simulink model "WF_offshore"  (R2024a)
settings: Solver=VariableStepAuto  StartTime=0  StopTime=1  RelTol=1e-3
values from neighbouring files (symbols this model uses):
  c_c = 0.177e-6    (= 1.77e-07)    [WF_onshore_SSO_GFL.m]    (also in WF_physical_param_offshore_supersynchronous.m = cable_220(i,6)*1e-9; WF_physical_param_onshore_SSO_020625.m = cable_220(i,6)*1e-9; initialize_params_agg.m)
  c_c_eff = c_c*n_cables    [WF_onshore_SSO_GFL.m]    (also in WF_physical_param_offshore_supersynchronous.m; WF_physical_param_onshore_SSO_020625.m; initialize_params_agg.m)
  cvtr = initialize_NR_VSC_GF(cvtr)    [NR_steadystate_VSC_GF.m]    (also in WF_onshore_SSO_GFL.m = setfield(cvtr,'parameters', p_vary.name,p_vary.val(i)); WF_physical_param_offshore_supersynchronous.m = setfield(cvtr,'parameters', p_vary.name,p_vary.val(i)); WF_physical_param_onshore_SSO_020625.m = setfield(cvtr,'parameters', p_vary.name,p_vary.val(i)); impedance_WT_blackbox.m = base_values(cvtr))
  D_C = 10:4:100    [WF_onshore_SSO_GFL.m]    (also in WF_parameter_variation.m = 10:4:150; WF_physical_param.m = 10:4:150; WF_physical_param_offshore_supersynchronous.m = 50; WF_physical_param_onshore_SSO_020625.m = 50)
  enable_pll = 1    [impedance_WT_agg.m]    (also in initialize_WT_agg.m; initialize_WT_default_gfl.m; initialize_WT_default_offshore_super.m)
  f1 = 50    [WF_onshore_SSO_GFL.m]    (also in WF_physical_param_offshore_supersynchronous.m; WF_physical_param_onshore_SSO_020625.m; initialize_params_agg.m)
  i = 1    [WF_physical_param_offshore_supersynchronous.m]    (also in WF_physical_param_onshore_SSO_020625.m)
  L = inv(R)    [participation_factors_VSC_GF.m]
  l_c = 0.386e-3    (= 0.000386)    [WF_onshore_SSO_GFL.m]    (also in WF_physical_param_offshore_supersynchronous.m = cable_220(i,5)*1e-3; WF_physical_param_onshore_SSO_020625.m = cable_220(i,5)*1e-3; initialize_params_agg.m)
  l_c_eff = l_c/n_cables    [WF_onshore_SSO_GFL.m]    (also in WF_physical_param_offshore_supersynchronous.m; WF_physical_param_onshore_SSO_020625.m; initialize_params_agg.m)
  L_comp = sqrt(2)*l_comp*(Z_b_G/(2*pi*f1))    [WF_physical_param.m]    (also in WF_physical_param_offshore_supersynchronous.m = sqrt(2)*((1/(c_c_eff/2*D_C*2*pi*f1))-(l_tf_wf*(Z_b_G)+(l_c_e; WF_physical_param_onshore_SSO_020625.m = sqrt(2)*((1/(c_c_eff/2*D_C*2*pi*f1))-(l_tf_wf*(Z_b_G)+(l_c_e; initialize_params_agg.m)
  l_OH = 0.2    [WF_onshore_SSO_GFL.m]    (also in WF_physical_param_offshore_supersynchronous.m = 0.1; WF_physical_param_onshore_SSO_020625.m = 0.1; initialize_params_agg.m = 0.1)
  l_tf_wf = tf_params(2,2)    [IM_WF_agg.m]    (also in WF_onshore_SSO_GFL.m = 0.05; WF_physical_param_offshore_supersynchronous.m = 0.05; WF_physical_param_onshore_SSO_020625.m = 0.05; initialize_params_agg.m = 0.05)
  l_tf_wt = tf_params(1,2)    [IM_WF_agg.m]    (also in WF_onshore_SSO_GFL.m = 0.0392; WF_physical_param_offshore_supersynchronous.m = 0.0392; WF_physical_param_onshore_SSO_020625.m = 0.0392; initialize_params_agg.m = 0.0392)
  Lg = p_vary(i)*((Z_b_G/(2*pi*f1)))    [WF_onshore_SSO_GFL.m]    (also in WF_physical_param_offshore_supersynchronous.m; WF_physical_param_onshore_SSO_020625.m; initialize_params_agg.m = 0.1*((Z_b_G/(2*pi*f1))))
  Lg1 = Lg    [WF_physical_param_offshore_supersynchronous.m]    (also in WF_physical_param_onshore_SSO_020625.m)
  Lg2 = Lg    [WF_physical_param_offshore_supersynchronous.m]    (also in WF_physical_param_onshore_SSO_020625.m)
  r_c = 27e-3    (= 0.027)    [WF_onshore_SSO_GFL.m]    (also in WF_physical_param_offshore_supersynchronous.m = cable_220(i,4)*1e-3; WF_physical_param_onshore_SSO_020625.m = cable_220(i,4)*1e-3; initialize_params_agg.m)
  r_c_eff = r_c/n_cables    [WF_onshore_SSO_GFL.m]    (also in WF_physical_param_offshore_supersynchronous.m; WF_physical_param_onshore_SSO_020625.m; initialize_params_agg.m)
  r_diss = .1    (= 0.1)    [WF_physical_param_offshore_supersynchronous.m]    (also in WF_physical_param_onshore_SSO_020625.m; calculate_WF.m; initialize_params_agg.m)
  r_OH = 0.02    [WF_onshore_SSO_GFL.m]    (also in WF_physical_param_offshore_supersynchronous.m = 0.01; WF_physical_param_onshore_SSO_020625.m = 0.01; initialize_params_agg.m)
  r_tf_wf = tf_params(2,1)    [IM_WF_agg.m]    (also in WF_onshore_SSO_GFL.m = 0.005; WF_physical_param_offshore_supersynchronous.m = 0.005; WF_physical_param_onshore_SSO_020625.m = 0.005; initialize_params_agg.m = 0.005)
  r_tf_wt = tf_params(1,1)    [IM_WF_agg.m]    (also in WF_onshore_SSO_GFL.m = 0.0056; WF_physical_param_offshore_supersynchronous.m = 0.0056; WF_physical_param_onshore_SSO_020625.m = 0.0056; initialize_params_agg.m = 0.0056)
  Rg = rg*Z_b_G    [WF_onshore_SSO_GFL.m]    (also in WF_physical_param_offshore_supersynchronous.m; WF_physical_param_onshore_SSO_020625.m; initialize_params_agg.m = 0.01*Z_b_G)
  Sb_WF = (3*1)*5e6    (= 15000000)    [WF_onshore_SSO_GFL.m]    (also in WF_physical_param_offshore_supersynchronous.m; WF_physical_param_onshore_SSO_020625.m; impedance_WT_blackbox.m = n_t*Sb_WT; initialize_params_agg.m = 1000000000)
  Sb_WT = 5e6    (= 5000000)    [IM_WF.m]    (also in WF_onshore_SSO_GFL.m; WF_physical_param_offshore_supersynchronous.m; WF_physical_param_onshore_SSO_020625.m; initialize_params_agg.m)
  selector_current_reference = 3    [impedance_WT_agg.m]    (also in initialize_WT_agg.m; initialize_WT_default_gfl.m; initialize_WT_default_offshore_super.m)
  selector_omega_reference = 1    [impedance_WT_agg.m]    (also in initialize_WT_agg.m; initialize_WT_default_gfl.m; initialize_WT_default_offshore_super.m)
  V_coll = 33e3    (= 33000)    [WF_onshore_SSO_GFL.m]    (also in WF_physical_param_offshore_supersynchronous.m; WF_physical_param_onshore_SSO_020625.m; initialize_params_agg.m)
  V_trans = 220e3    (= 220000)    [WF_onshore_SSO_GFL.m]    (also in WF_physical_param_offshore_supersynchronous.m; WF_physical_param_onshore_SSO_020625.m; initialize_params_agg.m)
  Z_b_G = (V_trans/sqrt(3/2))^2/Sb_WF    [WF_onshore_SSO_GFL.m]    (also in WF_physical_param_offshore_supersynchronous.m = (V_b_trans)^2/Sb_WF; WF_physical_param_onshore_SSO_020625.m = (V_b_trans)^2/Sb_WF; initialize_params_agg.m = (V_b_trans)^2/Sb_WF)
undefined symbols (not defined in the file or in its folder): opts, R
libraries: spsSeriesRLCBranchLib x105, simulink_extras x104, simulink x52, spsThreePhaseVIMeasurementLib x42, spsControlledVoltageSourceLib x42, spsGroundLib x41, spsThreePhaseTransformerTwoWindingsLib x14, powerlib_extras x13, spsVariableInductorLib x9, spsIdealSwitchLib x6, spsVariableCapacitorLib x6, spsThreePhaseSeriesRLCBranchLib x4
(part 13 of 13)

== system WF_offshore/WT_MF4/Control System/Current controller/Subsystem1 ==
  in : Inport
  Demux : Demux  Outputs=2
  Mux : Mux  Inputs=2
  Subsystem3 : Subsystem
  Subsystem6 : Subsystem
  Transfer Fcn (with initial outputs) : simulink_extras/Additional Linear/Transfer Fcn (with initial outputs)  N=[Omega]  D="[1  Omega]"  Y0=xd0  U0=xd0
  Transfer Fcn (with initial outputs)1 : simulink_extras/Additional Linear/Transfer Fcn (with initial outputs)  N=[Omega]  D="[1  Omega]"  Y0=xq0  U0=xq0
  out : Outport
  wires:
  Demux/2 -> Transfer Fcn (with initial outputs)1/1
  Demux/1 -> Transfer Fcn (with initial outputs)/1
  Subsystem3/1(x_d+ix_q) -> out/1
  in/1 -> Subsystem6/1(x_d+ix_q)
  Subsystem6/1(x_dq) -> Demux/1
  Mux/1 -> Subsystem3/1(x_dq)
  Transfer Fcn (with initial outputs)1/1 -> Mux/2
  Transfer Fcn (with initial outputs)/1 -> Mux/1

== system WF_offshore/WT_MF4/Control System/PLL1/Subsystem1 ==
  x_d+ix_q : Inport
  Complex to Real-Imag2 : ComplexToRealImag
  Mux : Mux  Inputs=2
  x_dq : Outport
  wires:
  Complex to Real-Imag2/1 -> Mux/1
  Complex to Real-Imag2/2 -> Mux/2
  Mux/1 -> x_dq/1
  x_d+ix_q/1 -> Complex to Real-Imag2/1

== system WF_offshore/WT_MF4/Control System/PLL1/Subsystem3 ==
  x_dq : Inport
  Demux : Demux  Outputs=2
  Real-Imag to Complex : RealImagToComplex
  x_d+ix_q : Outport
  wires:
  Real-Imag to Complex/1 -> x_d+ix_q/1
  x_dq/1 -> Demux/1
  Demux/2 -> Real-Imag to Complex/2
  Demux/1 -> Real-Imag to Complex/1

== system WF_offshore/WT_MF4/Control System/PQ controller/Subsystem3 ==
  x_dq : Inport
  Demux : Demux  Outputs=2
  Real-Imag to Complex : RealImagToComplex
  x_d+ix_q : Outport
  wires:
  Real-Imag to Complex/1 -> x_d+ix_q/1
  x_dq/1 -> Demux/1
  Demux/2 -> Real-Imag to Complex/2
  Demux/1 -> Real-Imag to Complex/1

== system WF_offshore/WT_MF4/Control System/Voltage controller DEM/Subsystem ==
  x : Inport
  x0 : Inport  Port=2
  Complex to Real-Imag : ComplexToRealImag
  Complex to Real-Imag1 : ComplexToRealImag
  Integrator : Integrator  InitialConditionSource=external
  Integrator1 : Integrator  InitialConditionSource=external
  Real-Imag to Complex : RealImagToComplex
  x/s : Outport
  wires:
  Integrator/1 -> Real-Imag to Complex/2
  Integrator1/1 -> Real-Imag to Complex/1
  x0/1 -> Complex to Real-Imag1/1
  Real-Imag to Complex/1 -> x/s/1
  x/1 -> Complex to Real-Imag/1
  Complex to Real-Imag1/2 -> Integrator/2
  Complex to Real-Imag1/1 -> Integrator1/2
  Complex to Real-Imag/2 -> Integrator/1
  Complex to Real-Imag/1 -> Integrator1/1

== system WF_offshore/WT_MF4/Control System/Voltage controller QSEM/Subsystem2 ==
  x_d+ix_q : Inport
  Complex to Real-Imag2 : ComplexToRealImag
  Mux : Mux  Inputs=2
  x_dq : Outport
  wires:
  Complex to Real-Imag2/1 -> Mux/1
  Complex to Real-Imag2/2 -> Mux/2
  Mux/1 -> x_dq/1
  x_d+ix_q/1 -> Complex to Real-Imag2/1

== system WF_offshore/WT_MF4/Control System/Voltage controller QSEM/Subsystem3 ==
  x_dq : Inport
  Demux : Demux  Outputs=2
  Real-Imag to Complex : RealImagToComplex
  x_d+ix_q : Outport
  wires:
  Real-Imag to Complex/1 -> x_d+ix_q/1
  x_dq/1 -> Demux/1
  Demux/2 -> Real-Imag to Complex/2
  Demux/1 -> Real-Imag to Complex/1

== system WF_offshore/WT_MF4/Control System/Voltage controller VCVSM/Subsystem ==
  x : Inport
  x0 : Inport  Port=2
  Complex to Real-Imag : ComplexToRealImag
  Complex to Real-Imag1 : ComplexToRealImag
  Integrator : Integrator  InitialConditionSource=external
  Integrator1 : Integrator  InitialConditionSource=external
  Real-Imag to Complex : RealImagToComplex
  x/s : Outport
  wires:
  Integrator/1 -> Real-Imag to Complex/2
  Integrator1/1 -> Real-Imag to Complex/1
  x0/1 -> Complex to Real-Imag1/1
  Real-Imag to Complex/1 -> x/s/1
  x/1 -> Complex to Real-Imag/1
  Complex to Real-Imag1/2 -> Integrator/2
  Complex to Real-Imag1/1 -> Integrator1/2
  Complex to Real-Imag/2 -> Integrator/1
  Complex to Real-Imag/1 -> Integrator1/1

== system WF_offshore/WT_MF5/Control System/Current controller/Subsystem ==
  x : Inport
  x0 : Inport  Port=2
  Complex to Real-Imag : ComplexToRealImag
  Complex to Real-Imag1 : ComplexToRealImag
  Integrator : Integrator  InitialConditionSource=external  AbsoluteTolerance=1e-10
  Integrator1 : Integrator  InitialConditionSource=external  AbsoluteTolerance=1e-15
  Real-Imag to Complex : RealImagToComplex
  x/s : Outport
  wires:
  Complex to Real-Imag/1 -> Integrator/1
  Complex to Real-Imag1/1 -> Integrator/2
  Complex to Real-Imag1/2 -> Integrator1/2
  x/1 -> Complex to Real-Imag/1
  Real-Imag to Complex/1 -> x/s/1
  x0/1 -> Complex to Real-Imag1/1
  Integrator1/1 -> Real-Imag to Complex/2
  Integrator/1 -> Real-Imag to Complex/1
  Complex to Real-Imag/2 -> Integrator1/1

== system WF_offshore/WT_MF5/Control System/Current controller/Subsystem1 ==
  in : Inport
  Demux : Demux  Outputs=2
  Mux : Mux  Inputs=2
  Subsystem3 : Subsystem
  Subsystem6 : Subsystem
  Transfer Fcn (with initial outputs) : simulink_extras/Additional Linear/Transfer Fcn (with initial outputs)  N=[Omega]  D="[1  Omega]"  Y0=xd0  U0=xd0
  Transfer Fcn (with initial outputs)1 : simulink_extras/Additional Linear/Transfer Fcn (with initial outputs)  N=[Omega]  D="[1  Omega]"  Y0=xq0  U0=xq0
  out : Outport
  wires:
  Transfer Fcn (with initial outputs)/1 -> Mux/1
  Transfer Fcn (with initial outputs)1/1 -> Mux/2
  Mux/1 -> Subsystem3/1(x_dq)
  Subsystem6/1(x_dq) -> Demux/1
  in/1 -> Subsystem6/1(x_d+ix_q)
  Subsystem3/1(x_d+ix_q) -> out/1
  Demux/1 -> Transfer Fcn (with initial outputs)/1
  Demux/2 -> Transfer Fcn (with initial outputs)1/1

== system WF_offshore/WT_MF5/Control System/PLL1/Subsystem1 ==
  x_d+ix_q : Inport
  Complex to Real-Imag2 : ComplexToRealImag
  Mux : Mux  Inputs=2
  x_dq : Outport
  wires:
  x_d+ix_q/1 -> Complex to Real-Imag2/1
  Mux/1 -> x_dq/1
  Complex to Real-Imag2/2 -> Mux/2
  Complex to Real-Imag2/1 -> Mux/1

== system WF_offshore/WT_MF5/Control System/PLL1/Subsystem3 ==
  x_dq : Inport
  Demux : Demux  Outputs=2
  Real-Imag to Complex : RealImagToComplex
  x_d+ix_q : Outport
  wires:
  Demux/1 -> Real-Imag to Complex/1
  Demux/2 -> Real-Imag to Complex/2
  x_dq/1 -> Demux/1
  Real-Imag to Complex/1 -> x_d+ix_q/1

== system WF_offshore/WT_MF5/Control System/PQ controller/Subsystem3 ==
  x_dq : Inport
  Demux : Demux  Outputs=2
  Real-Imag to Complex : RealImagToComplex
  x_d+ix_q : Outport
  wires:
  Demux/1 -> Real-Imag to Complex/1
  Demux/2 -> Real-Imag to Complex/2
  x_dq/1 -> Demux/1
  Real-Imag to Complex/1 -> x_d+ix_q/1

== system WF_offshore/WT_MF5/Control System/Voltage controller DEM/Subsystem ==
  x : Inport
  x0 : Inport  Port=2
  Complex to Real-Imag : ComplexToRealImag
  Complex to Real-Imag1 : ComplexToRealImag
  Integrator : Integrator  InitialConditionSource=external
  Integrator1 : Integrator  InitialConditionSource=external
  Real-Imag to Complex : RealImagToComplex
  x/s : Outport
  wires:
  Complex to Real-Imag/1 -> Integrator1/1
  Complex to Real-Imag/2 -> Integrator/1
  Complex to Real-Imag1/1 -> Integrator1/2
  Complex to Real-Imag1/2 -> Integrator/2
  x/1 -> Complex to Real-Imag/1
  Real-Imag to Complex/1 -> x/s/1
  x0/1 -> Complex to Real-Imag1/1
  Integrator1/1 -> Real-Imag to Complex/1
  Integrator/1 -> Real-Imag to Complex/2

== system WF_offshore/WT_MF5/Control System/Voltage controller QSEM/Subsystem2 ==
  x_d+ix_q : Inport
  Complex to Real-Imag2 : ComplexToRealImag
  Mux : Mux  Inputs=2
  x_dq : Outport
  wires:
  x_d+ix_q/1 -> Complex to Real-Imag2/1
  Mux/1 -> x_dq/1
  Complex to Real-Imag2/2 -> Mux/2
  Complex to Real-Imag2/1 -> Mux/1

== system WF_offshore/WT_MF5/Control System/Voltage controller QSEM/Subsystem3 ==
  x_dq : Inport
  Demux : Demux  Outputs=2
  Real-Imag to Complex : RealImagToComplex
  x_d+ix_q : Outport
  wires:
  Demux/1 -> Real-Imag to Complex/1
  Demux/2 -> Real-Imag to Complex/2
  x_dq/1 -> Demux/1
  Real-Imag to Complex/1 -> x_d+ix_q/1

== system WF_offshore/WT_MF5/Control System/Voltage controller VCVSM/Subsystem ==
  x : Inport
  x0 : Inport  Port=2
  Complex to Real-Imag : ComplexToRealImag
  Complex to Real-Imag1 : ComplexToRealImag
  Integrator : Integrator  InitialConditionSource=external
  Integrator1 : Integrator  InitialConditionSource=external
  Real-Imag to Complex : RealImagToComplex
  x/s : Outport
  wires:
  Complex to Real-Imag/1 -> Integrator1/1
  Complex to Real-Imag/2 -> Integrator/1
  Complex to Real-Imag1/1 -> Integrator1/2
  Complex to Real-Imag1/2 -> Integrator/2
  x/1 -> Complex to Real-Imag/1
  Real-Imag to Complex/1 -> x/s/1
  x0/1 -> Complex to Real-Imag1/1
  Integrator1/1 -> Real-Imag to Complex/1
  Integrator/1 -> Real-Imag to Complex/2

== system WF_offshore/WT_MF6/Control System/Current controller/Subsystem ==
  x : Inport
  x0 : Inport  Port=2
  Complex to Real-Imag : ComplexToRealImag
  Complex to Real-Imag1 : ComplexToRealImag
  Integrator : Integrator  InitialConditionSource=external  AbsoluteTolerance=1e-10
  Integrator1 : Integrator  InitialConditionSource=external  AbsoluteTolerance=1e-15
  Real-Imag to Complex : RealImagToComplex
  x/s : Outport
  wires:
  Complex to Real-Imag/2 -> Integrator1/1
  Integrator/1 -> Real-Imag to Complex/1
  Integrator1/1 -> Real-Imag to Complex/2
  x0/1 -> Complex to Real-Imag1/1
  Real-Imag to Complex/1 -> x/s/1
  x/1 -> Complex to Real-Imag/1
  Complex to Real-Imag1/2 -> Integrator1/2
  Complex to Real-Imag1/1 -> Integrator/2
  Complex to Real-Imag/1 -> Integrator/1

== system WF_offshore/WT_MF6/Control System/Current controller/Subsystem1 ==
  in : Inport
  Demux : Demux  Outputs=2
  Mux : Mux  Inputs=2
  Subsystem3 : Subsystem
  Subsystem6 : Subsystem
  Transfer Fcn (with initial outputs) : simulink_extras/Additional Linear/Transfer Fcn (with initial outputs)  N=[Omega]  D="[1  Omega]"  Y0=xd0  U0=xd0
  Transfer Fcn (with initial outputs)1 : simulink_extras/Additional Linear/Transfer Fcn (with initial outputs)  N=[Omega]  D="[1  Omega]"  Y0=xq0  U0=xq0
  out : Outport
  wires:
  Demux/2 -> Transfer Fcn (with initial outputs)1/1
  Demux/1 -> Transfer Fcn (with initial outputs)/1
  Subsystem3/1(x_d+ix_q) -> out/1
  in/1 -> Subsystem6/1(x_d+ix_q)
  Subsystem6/1(x_dq) -> Demux/1
  Mux/1 -> Subsystem3/1(x_dq)
  Transfer Fcn (with initial outputs)1/1 -> Mux/2
  Transfer Fcn (with initial outputs)/1 -> Mux/1

== system WF_offshore/WT_MF6/Control System/PLL1/Subsystem1 ==
  x_d+ix_q : Inport
  Complex to Real-Imag2 : ComplexToRealImag
  Mux : Mux  Inputs=2
  x_dq : Outport
  wires:
  Complex to Real-Imag2/1 -> Mux/1
  Complex to Real-Imag2/2 -> Mux/2
  Mux/1 -> x_dq/1
  x_d+ix_q/1 -> Complex to Real-Imag2/1

== system WF_offshore/WT_MF6/Control System/PLL1/Subsystem3 ==
  x_dq : Inport
  Demux : Demux  Outputs=2
  Real-Imag to Complex : RealImagToComplex
  x_d+ix_q : Outport
  wires:
  Real-Imag to Complex/1 -> x_d+ix_q/1
  x_dq/1 -> Demux/1
  Demux/2 -> Real-Imag to Complex/2
  Demux/1 -> Real-Imag to Complex/1

== system WF_offshore/WT_MF6/Control System/PQ controller/Subsystem3 ==
  x_dq : Inport
  Demux : Demux  Outputs=2
  Real-Imag to Complex : RealImagToComplex
  x_d+ix_q : Outport
  wires:
  Real-Imag to Complex/1 -> x_d+ix_q/1
  x_dq/1 -> Demux/1
  Demux/2 -> Real-Imag to Complex/2
  Demux/1 -> Real-Imag to Complex/1

== system WF_offshore/WT_MF6/Control System/Voltage controller DEM/Subsystem ==
  x : Inport
  x0 : Inport  Port=2
  Complex to Real-Imag : ComplexToRealImag
  Complex to Real-Imag1 : ComplexToRealImag
  Integrator : Integrator  InitialConditionSource=external
  Integrator1 : Integrator  InitialConditionSource=external
  Real-Imag to Complex : RealImagToComplex
  x/s : Outport
  wires:
  Integrator/1 -> Real-Imag to Complex/2
  Integrator1/1 -> Real-Imag to Complex/1
  x0/1 -> Complex to Real-Imag1/1
  Real-Imag to Complex/1 -> x/s/1
  x/1 -> Complex to Real-Imag/1
  Complex to Real-Imag1/2 -> Integrator/2
  Complex to Real-Imag1/1 -> Integrator1/2
  Complex to Real-Imag/2 -> Integrator/1
  Complex to Real-Imag/1 -> Integrator1/1

== system WF_offshore/WT_MF6/Control System/Voltage controller QSEM/Subsystem2 ==
  x_d+ix_q : Inport
  Complex to Real-Imag2 : ComplexToRealImag
  Mux : Mux  Inputs=2
  x_dq : Outport
  wires:
  Complex to Real-Imag2/1 -> Mux/1
  Complex to Real-Imag2/2 -> Mux/2
  Mux/1 -> x_dq/1
  x_d+ix_q/1 -> Complex to Real-Imag2/1

== system WF_offshore/WT_MF6/Control System/Voltage controller QSEM/Subsystem3 ==
  x_dq : Inport
  Demux : Demux  Outputs=2
  Real-Imag to Complex : RealImagToComplex
  x_d+ix_q : Outport
  wires:
  Real-Imag to Complex/1 -> x_d+ix_q/1
  x_dq/1 -> Demux/1
  Demux/2 -> Real-Imag to Complex/2
  Demux/1 -> Real-Imag to Complex/1

== system WF_offshore/WT_MF6/Control System/Voltage controller VCVSM/Subsystem ==
  x : Inport
  x0 : Inport  Port=2
  Complex to Real-Imag : ComplexToRealImag
  Complex to Real-Imag1 : ComplexToRealImag
  Integrator : Integrator  InitialConditionSource=external
  Integrator1 : Integrator  InitialConditionSource=external
  Real-Imag to Complex : RealImagToComplex
  x/s : Outport
  wires:
  Integrator/1 -> Real-Imag to Complex/2
  Integrator1/1 -> Real-Imag to Complex/1
  x0/1 -> Complex to Real-Imag1/1
  Real-Imag to Complex/1 -> x/s/1
  x/1 -> Complex to Real-Imag/1
  Complex to Real-Imag1/2 -> Integrator/2
  Complex to Real-Imag1/1 -> Integrator1/2
  Complex to Real-Imag/2 -> Integrator/1
  Complex to Real-Imag/1 -> Integrator1/1

== system WF_offshore/WT_MF7/Control System/Current controller/Subsystem ==
  x : Inport
  x0 : Inport  Port=2
  Complex to Real-Imag : ComplexToRealImag
  Complex to Real-Imag1 : ComplexToRealImag
  Integrator : Integrator  InitialConditionSource=external  AbsoluteTolerance=1e-10
  Integrator1 : Integrator  InitialConditionSource=external  AbsoluteTolerance=1e-15
  Real-Imag to Complex : RealImagToComplex
  x/s : Outport
  wires:
  Complex to Real-Imag/1 -> Integrator/1
  Complex to Real-Imag1/1 -> Integrator/2
  Complex to Real-Imag1/2 -> Integrator1/2
  x/1 -> Complex to Real-Imag/1
  Real-Imag to Complex/1 -> x/s/1
  x0/1 -> Complex to Real-Imag1/1
  Integrator1/1 -> Real-Imag to Complex/2
  Integrator/1 -> Real-Imag to Complex/1
  Complex to Real-Imag/2 -> Integrator1/1

== system WF_offshore/WT_MF7/Control System/Current controller/Subsystem1 ==
  in : Inport
  Demux : Demux  Outputs=2
  Mux : Mux  Inputs=2
  Subsystem3 : Subsystem
  Subsystem6 : Subsystem
  Transfer Fcn (with initial outputs) : simulink_extras/Additional Linear/Transfer Fcn (with initial outputs)  N=[Omega]  D="[1  Omega]"  Y0=xd0  U0=xd0
  Transfer Fcn (with initial outputs)1 : simulink_extras/Additional Linear/Transfer Fcn (with initial outputs)  N=[Omega]  D="[1  Omega]"  Y0=xq0  U0=xq0
  out : Outport
  wires:
  Transfer Fcn (with initial outputs)/1 -> Mux/1
  Transfer Fcn (with initial outputs)1/1 -> Mux/2
  Mux/1 -> Subsystem3/1(x_dq)
  Subsystem6/1(x_dq) -> Demux/1
  in/1 -> Subsystem6/1(x_d+ix_q)
  Subsystem3/1(x_d+ix_q) -> out/1
  Demux/1 -> Transfer Fcn (with initial outputs)/1
  Demux/2 -> Transfer Fcn (with initial outputs)1/1

== system WF_offshore/WT_MF7/Control System/PLL1/Subsystem1 ==
  x_d+ix_q : Inport
  Complex to Real-Imag2 : ComplexToRealImag
  Mux : Mux  Inputs=2
  x_dq : Outport
  wires:
  x_d+ix_q/1 -> Complex to Real-Imag2/1
  Mux/1 -> x_dq/1
  Complex to Real-Imag2/2 -> Mux/2
  Complex to Real-Imag2/1 -> Mux/1

== system WF_offshore/WT_MF7/Control System/PLL1/Subsystem3 ==
  x_dq : Inport
  Demux : Demux  Outputs=2
  Real-Imag to Complex : RealImagToComplex
  x_d+ix_q : Outport
  wires:
  Demux/1 -> Real-Imag to Complex/1
  Demux/2 -> Real-Imag to Complex/2
  x_dq/1 -> Demux/1
  Real-Imag to Complex/1 -> x_d+ix_q/1

== system WF_offshore/WT_MF7/Control System/PQ controller/Subsystem3 ==
  x_dq : Inport
  Demux : Demux  Outputs=2
  Real-Imag to Complex : RealImagToComplex
  x_d+ix_q : Outport
  wires:
  Demux/1 -> Real-Imag to Complex/1
  Demux/2 -> Real-Imag to Complex/2
  x_dq/1 -> Demux/1
  Real-Imag to Complex/1 -> x_d+ix_q/1

== system WF_offshore/WT_MF7/Control System/Voltage controller DEM/Subsystem ==
  x : Inport
  x0 : Inport  Port=2
  Complex to Real-Imag : ComplexToRealImag
  Complex to Real-Imag1 : ComplexToRealImag
  Integrator : Integrator  InitialConditionSource=external
  Integrator1 : Integrator  InitialConditionSource=external
  Real-Imag to Complex : RealImagToComplex
  x/s : Outport
  wires:
  Complex to Real-Imag/1 -> Integrator1/1
  Complex to Real-Imag/2 -> Integrator/1
  Complex to Real-Imag1/1 -> Integrator1/2
  Complex to Real-Imag1/2 -> Integrator/2
  x/1 -> Complex to Real-Imag/1
  Real-Imag to Complex/1 -> x/s/1
  x0/1 -> Complex to Real-Imag1/1
  Integrator1/1 -> Real-Imag to Complex/1
  Integrator/1 -> Real-Imag to Complex/2

== system WF_offshore/WT_MF7/Control System/Voltage controller QSEM/Subsystem2 ==
  x_d+ix_q : Inport
  Complex to Real-Imag2 : ComplexToRealImag
  Mux : Mux  Inputs=2
  x_dq : Outport
  wires:
  x_d+ix_q/1 -> Complex to Real-Imag2/1
  Mux/1 -> x_dq/1
  Complex to Real-Imag2/2 -> Mux/2
  Complex to Real-Imag2/1 -> Mux/1

== system WF_offshore/WT_MF7/Control System/Voltage controller QSEM/Subsystem3 ==
  x_dq : Inport
  Demux : Demux  Outputs=2
  Real-Imag to Complex : RealImagToComplex
  x_d+ix_q : Outport
  wires:
  Demux/1 -> Real-Imag to Complex/1
  Demux/2 -> Real-Imag to Complex/2
  x_dq/1 -> Demux/1
  Real-Imag to Complex/1 -> x_d+ix_q/1

== system WF_offshore/WT_MF7/Control System/Voltage controller VCVSM/Subsystem ==
  x : Inport
  x0 : Inport  Port=2
  Complex to Real-Imag : ComplexToRealImag
  Complex to Real-Imag1 : ComplexToRealImag
  Integrator : Integrator  InitialConditionSource=external
  Integrator1 : Integrator  InitialConditionSource=external
  Real-Imag to Complex : RealImagToComplex
  x/s : Outport
  wires:
  Complex to Real-Imag/1 -> Integrator1/1
  Complex to Real-Imag/2 -> Integrator/1
  Complex to Real-Imag1/1 -> Integrator1/2
  Complex to Real-Imag1/2 -> Integrator/2
  x/1 -> Complex to Real-Imag/1
  Real-Imag to Complex/1 -> x/s/1
  x0/1 -> Complex to Real-Imag1/1
  Integrator1/1 -> Real-Imag to Complex/1
  Integrator/1 -> Real-Imag to Complex/2

== system WF_offshore/WT_MF8/Control System/Current controller/Subsystem ==
  x : Inport
  x0 : Inport  Port=2
  Complex to Real-Imag : ComplexToRealImag
  Complex to Real-Imag1 : ComplexToRealImag
  Integrator : Integrator  InitialConditionSource=external  AbsoluteTolerance=1e-10
  Integrator1 : Integrator  InitialConditionSource=external  AbsoluteTolerance=1e-15
  Real-Imag to Complex : RealImagToComplex
  x/s : Outport
  wires:
  Complex to Real-Imag/2 -> Integrator1/1
  Integrator/1 -> Real-Imag to Complex/1
  Integrator1/1 -> Real-Imag to Complex/2
  x0/1 -> Complex to Real-Imag1/1
  Real-Imag to Complex/1 -> x/s/1
  x/1 -> Complex to Real-Imag/1
  Complex to Real-Imag1/2 -> Integrator1/2
  Complex to Real-Imag1/1 -> Integrator/2
  Complex to Real-Imag/1 -> Integrator/1

== system WF_offshore/WT_MF8/Control System/Current controller/Subsystem1 ==
  in : Inport
  Demux : Demux  Outputs=2
  Mux : Mux  Inputs=2
  Subsystem3 : Subsystem
  Subsystem6 : Subsystem
  Transfer Fcn (with initial outputs) : simulink_extras/Additional Linear/Transfer Fcn (with initial outputs)  N=[Omega]  D="[1  Omega]"  Y0=xd0  U0=xd0
  Transfer Fcn (with initial outputs)1 : simulink_extras/Additional Linear/Transfer Fcn (with initial outputs)  N=[Omega]  D="[1  Omega]"  Y0=xq0  U0=xq0
  out : Outport
  wires:
  Demux/2 -> Transfer Fcn (with initial outputs)1/1
  Demux/1 -> Transfer Fcn (with initial outputs)/1
  Subsystem3/1(x_d+ix_q) -> out/1
  in/1 -> Subsystem6/1(x_d+ix_q)
  Subsystem6/1(x_dq) -> Demux/1
  Mux/1 -> Subsystem3/1(x_dq)
  Transfer Fcn (with initial outputs)1/1 -> Mux/2
  Transfer Fcn (with initial outputs)/1 -> Mux/1

== system WF_offshore/WT_MF8/Control System/PLL1/Subsystem1 ==
  x_d+ix_q : Inport
  Complex to Real-Imag2 : ComplexToRealImag
  Mux : Mux  Inputs=2
  x_dq : Outport
  wires:
  Complex to Real-Imag2/1 -> Mux/1
  Complex to Real-Imag2/2 -> Mux/2
  Mux/1 -> x_dq/1
  x_d+ix_q/1 -> Complex to Real-Imag2/1

== system WF_offshore/WT_MF8/Control System/PLL1/Subsystem3 ==
  x_dq : Inport
  Demux : Demux  Outputs=2
  Real-Imag to Complex : RealImagToComplex
  x_d+ix_q : Outport
  wires:
  Real-Imag to Complex/1 -> x_d+ix_q/1
  x_dq/1 -> Demux/1
  Demux/2 -> Real-Imag to Complex/2
  Demux/1 -> Real-Imag to Complex/1

== system WF_offshore/WT_MF8/Control System/PQ controller/Subsystem3 ==
  x_dq : Inport
  Demux : Demux  Outputs=2
  Real-Imag to Complex : RealImagToComplex
  x_d+ix_q : Outport
  wires:
  Real-Imag to Complex/1 -> x_d+ix_q/1
  x_dq/1 -> Demux/1
  Demux/2 -> Real-Imag to Complex/2
  Demux/1 -> Real-Imag to Complex/1

== system WF_offshore/WT_MF8/Control System/Voltage controller DEM/Subsystem ==
  x : Inport
  x0 : Inport  Port=2
  Complex to Real-Imag : ComplexToRealImag
  Complex to Real-Imag1 : ComplexToRealImag
  Integrator : Integrator  InitialConditionSource=external
  Integrator1 : Integrator  InitialConditionSource=external
  Real-Imag to Complex : RealImagToComplex
  x/s : Outport
  wires:
  Integrator/1 -> Real-Imag to Complex/2
  Integrator1/1 -> Real-Imag to Complex/1
  x0/1 -> Complex to Real-Imag1/1
  Real-Imag to Complex/1 -> x/s/1
  x/1 -> Complex to Real-Imag/1
  Complex to Real-Imag1/2 -> Integrator/2
  Complex to Real-Imag1/1 -> Integrator1/2
  Complex to Real-Imag/2 -> Integrator/1
  Complex to Real-Imag/1 -> Integrator1/1

== system WF_offshore/WT_MF8/Control System/Voltage controller QSEM/Subsystem2 ==
  x_d+ix_q : Inport
  Complex to Real-Imag2 : ComplexToRealImag
  Mux : Mux  Inputs=2
  x_dq : Outport
  wires:
  Complex to Real-Imag2/1 -> Mux/1
  Complex to Real-Imag2/2 -> Mux/2
  Mux/1 -> x_dq/1
  x_d+ix_q/1 -> Complex to Real-Imag2/1

== system WF_offshore/WT_MF8/Control System/Voltage controller QSEM/Subsystem3 ==
  x_dq : Inport
  Demux : Demux  Outputs=2
  Real-Imag to Complex : RealImagToComplex
  x_d+ix_q : Outport
  wires:
  Real-Imag to Complex/1 -> x_d+ix_q/1
  x_dq/1 -> Demux/1
  Demux/2 -> Real-Imag to Complex/2
  Demux/1 -> Real-Imag to Complex/1

== system WF_offshore/WT_MF8/Control System/Voltage controller VCVSM/Subsystem ==
  x : Inport
  x0 : Inport  Port=2
  Complex to Real-Imag : ComplexToRealImag
  Complex to Real-Imag1 : ComplexToRealImag
  Integrator : Integrator  InitialConditionSource=external
  Integrator1 : Integrator  InitialConditionSource=external
  Real-Imag to Complex : RealImagToComplex
  x/s : Outport
  wires:
  Integrator/1 -> Real-Imag to Complex/2
  Integrator1/1 -> Real-Imag to Complex/1
  x0/1 -> Complex to Real-Imag1/1
  Real-Imag to Complex/1 -> x/s/1
  x/1 -> Complex to Real-Imag/1
  Complex to Real-Imag1/2 -> Integrator/2
  Complex to Real-Imag1/1 -> Integrator1/2
  Complex to Real-Imag/2 -> Integrator/1
  Complex to Real-Imag/1 -> Integrator1/1

== system WF_offshore/WT_MF9/Control System/Current controller/Subsystem ==
  x : Inport
  x0 : Inport  Port=2
  Complex to Real-Imag : ComplexToRealImag
  Complex to Real-Imag1 : ComplexToRealImag
  Integrator : Integrator  InitialConditionSource=external  AbsoluteTolerance=1e-10
  Integrator1 : Integrator  InitialConditionSource=external  AbsoluteTolerance=1e-15
  Real-Imag to Complex : RealImagToComplex
  x/s : Outport
  wires:
  Complex to Real-Imag/1 -> Integrator/1
  Complex to Real-Imag1/1 -> Integrator/2
  Complex to Real-Imag1/2 -> Integrator1/2
  x/1 -> Complex to Real-Imag/1
  Real-Imag to Complex/1 -> x/s/1
  x0/1 -> Complex to Real-Imag1/1
  Integrator1/1 -> Real-Imag to Complex/2
  Integrator/1 -> Real-Imag to Complex/1
  Complex to Real-Imag/2 -> Integrator1/1

== system WF_offshore/WT_MF9/Control System/Current controller/Subsystem1 ==
  in : Inport
  Demux : Demux  Outputs=2
  Mux : Mux  Inputs=2
  Subsystem3 : Subsystem
  Subsystem6 : Subsystem
  Transfer Fcn (with initial outputs) : simulink_extras/Additional Linear/Transfer Fcn (with initial outputs)  N=[Omega]  D="[1  Omega]"  Y0=xd0  U0=xd0
  Transfer Fcn (with initial outputs)1 : simulink_extras/Additional Linear/Transfer Fcn (with initial outputs)  N=[Omega]  D="[1  Omega]"  Y0=xq0  U0=xq0
  out : Outport
  wires:
  Transfer Fcn (with initial outputs)/1 -> Mux/1
  Transfer Fcn (with initial outputs)1/1 -> Mux/2
  Mux/1 -> Subsystem3/1(x_dq)
  Subsystem6/1(x_dq) -> Demux/1
  in/1 -> Subsystem6/1(x_d+ix_q)
  Subsystem3/1(x_d+ix_q) -> out/1
  Demux/1 -> Transfer Fcn (with initial outputs)/1
  Demux/2 -> Transfer Fcn (with initial outputs)1/1

== system WF_offshore/WT_MF9/Control System/PLL1/Subsystem1 ==
  x_d+ix_q : Inport
  Complex to Real-Imag2 : ComplexToRealImag
  Mux : Mux  Inputs=2
  x_dq : Outport
  wires:
  x_d+ix_q/1 -> Complex to Real-Imag2/1
  Mux/1 -> x_dq/1
  Complex to Real-Imag2/2 -> Mux/2
  Complex to Real-Imag2/1 -> Mux/1

== system WF_offshore/WT_MF9/Control System/PLL1/Subsystem3 ==
  x_dq : Inport
  Demux : Demux  Outputs=2
  Real-Imag to Complex : RealImagToComplex
  x_d+ix_q : Outport
  wires:
  Demux/1 -> Real-Imag to Complex/1
  Demux/2 -> Real-Imag to Complex/2
  x_dq/1 -> Demux/1
  Real-Imag to Complex/1 -> x_d+ix_q/1

== system WF_offshore/WT_MF9/Control System/PQ controller/Subsystem3 ==
  x_dq : Inport
  Demux : Demux  Outputs=2
  Real-Imag to Complex : RealImagToComplex
  x_d+ix_q : Outport
  wires:
  Demux/1 -> Real-Imag to Complex/1
  Demux/2 -> Real-Imag to Complex/2
  x_dq/1 -> Demux/1
  Real-Imag to Complex/1 -> x_d+ix_q/1

== system WF_offshore/WT_MF9/Control System/Voltage controller DEM/Subsystem ==
  x : Inport
  x0 : Inport  Port=2
  Complex to Real-Imag : ComplexToRealImag
  Complex to Real-Imag1 : ComplexToRealImag
  Integrator : Integrator  InitialConditionSource=external
  Integrator1 : Integrator  InitialConditionSource=external
  Real-Imag to Complex : RealImagToComplex
  x/s : Outport
  wires:
  Complex to Real-Imag/1 -> Integrator1/1
  Complex to Real-Imag/2 -> Integrator/1
  Complex to Real-Imag1/1 -> Integrator1/2
  Complex to Real-Imag1/2 -> Integrator/2
  x/1 -> Complex to Real-Imag/1
  Real-Imag to Complex/1 -> x/s/1
  x0/1 -> Complex to Real-Imag1/1
  Integrator1/1 -> Real-Imag to Complex/1
  Integrator/1 -> Real-Imag to Complex/2

== system WF_offshore/WT_MF9/Control System/Voltage controller QSEM/Subsystem2 ==
  x_d+ix_q : Inport
  Complex to Real-Imag2 : ComplexToRealImag
  Mux : Mux  Inputs=2
  x_dq : Outport
  wires:
  x_d+ix_q/1 -> Complex to Real-Imag2/1
  Mux/1 -> x_dq/1
  Complex to Real-Imag2/2 -> Mux/2
  Complex to Real-Imag2/1 -> Mux/1

== system WF_offshore/WT_MF9/Control System/Voltage controller QSEM/Subsystem3 ==
  x_dq : Inport
  Demux : Demux  Outputs=2
  Real-Imag to Complex : RealImagToComplex
  x_d+ix_q : Outport
  wires:
  Demux/1 -> Real-Imag to Complex/1
  Demux/2 -> Real-Imag to Complex/2
  x_dq/1 -> Demux/1
  Real-Imag to Complex/1 -> x_d+ix_q/1

== system WF_offshore/WT_MF9/Control System/Voltage controller VCVSM/Subsystem ==
  x : Inport
  x0 : Inport  Port=2
  Complex to Real-Imag : ComplexToRealImag
  Complex to Real-Imag1 : ComplexToRealImag
  Integrator : Integrator  InitialConditionSource=external
  Integrator1 : Integrator  InitialConditionSource=external
  Real-Imag to Complex : RealImagToComplex
  x/s : Outport
  wires:
  Complex to Real-Imag/1 -> Integrator1/1
  Complex to Real-Imag/2 -> Integrator/1
  Complex to Real-Imag1/1 -> Integrator1/2
  Complex to Real-Imag1/2 -> Integrator/2
  x/1 -> Complex to Real-Imag/1
  Real-Imag to Complex/1 -> x/s/1
  x0/1 -> Complex to Real-Imag1/1
  Integrator1/1 -> Real-Imag to Complex/1
  Integrator/1 -> Real-Imag to Complex/2

== system WF_offshore/WT_MF1/Control System/Current controller/Subsystem1/Subsystem3 ==
  x_dq : Inport
  Demux : Demux  Outputs=2
  Real-Imag to Complex : RealImagToComplex
  x_d+ix_q : Outport
  wires:
  Demux/1 -> Real-Imag to Complex/1
  Demux/2 -> Real-Imag to Complex/2
  x_dq/1 -> Demux/1
  Real-Imag to Complex/1 -> x_d+ix_q/1

== system WF_offshore/WT_MF1/Control System/Current controller/Subsystem1/Subsystem6 ==
  x_d+ix_q : Inport
  Complex to Real-Imag2 : ComplexToRealImag
  Mux : Mux  Inputs=2
  x_dq : Outport
  wires:
  Complex to Real-Imag2/1 -> Mux/1
  Complex to Real-Imag2/2 -> Mux/2
  Mux/1 -> x_dq/1
  x_d+ix_q/1 -> Complex to Real-Imag2/1

== system WF_offshore/WT_MF10/Control System/Current controller/Subsystem1/Subsystem3 ==
  x_dq : Inport
  Demux : Demux  Outputs=2
  Real-Imag to Complex : RealImagToComplex
  x_d+ix_q : Outport
  wires:
  Real-Imag to Complex/1 -> x_d+ix_q/1
  x_dq/1 -> Demux/1
  Demux/2 -> Real-Imag to Complex/2
  Demux/1 -> Real-Imag to Complex/1

== system WF_offshore/WT_MF10/Control System/Current controller/Subsystem1/Subsystem6 ==
  x_d+ix_q : Inport
  Complex to Real-Imag2 : ComplexToRealImag
  Mux : Mux  Inputs=2
  x_dq : Outport
  wires:
  x_d+ix_q/1 -> Complex to Real-Imag2/1
  Mux/1 -> x_dq/1
  Complex to Real-Imag2/2 -> Mux/2
  Complex to Real-Imag2/1 -> Mux/1

== system WF_offshore/WT_MF11/Control System/Current controller/Subsystem1/Subsystem3 ==
  x_dq : Inport
  Demux : Demux  Outputs=2
  Real-Imag to Complex : RealImagToComplex
  x_d+ix_q : Outport
  wires:
  Demux/1 -> Real-Imag to Complex/1
  Demux/2 -> Real-Imag to Complex/2
  x_dq/1 -> Demux/1
  Real-Imag to Complex/1 -> x_d+ix_q/1

== system WF_offshore/WT_MF11/Control System/Current controller/Subsystem1/Subsystem6 ==
  x_d+ix_q : Inport
  Complex to Real-Imag2 : ComplexToRealImag
  Mux : Mux  Inputs=2
  x_dq : Outport
  wires:
  Complex to Real-Imag2/1 -> Mux/1
  Complex to Real-Imag2/2 -> Mux/2
  Mux/1 -> x_dq/1
  x_d+ix_q/1 -> Complex to Real-Imag2/1

== system WF_offshore/WT_MF12/Control System/Current controller/Subsystem1/Subsystem3 ==
  x_dq : Inport
  Demux : Demux  Outputs=2
  Real-Imag to Complex : RealImagToComplex
  x_d+ix_q : Outport
  wires:
  Real-Imag to Complex/1 -> x_d+ix_q/1
  x_dq/1 -> Demux/1
  Demux/2 -> Real-Imag to Complex/2
  Demux/1 -> Real-Imag to Complex/1

== system WF_offshore/WT_MF12/Control System/Current controller/Subsystem1/Subsystem6 ==
  x_d+ix_q : Inport
  Complex to Real-Imag2 : ComplexToRealImag
  Mux : Mux  Inputs=2
  x_dq : Outport
  wires:
  x_d+ix_q/1 -> Complex to Real-Imag2/1
  Mux/1 -> x_dq/1
  Complex to Real-Imag2/2 -> Mux/2
  Complex to Real-Imag2/1 -> Mux/1

== system WF_offshore/WT_MF14/Control System/Current controller/Subsystem1/Subsystem3 ==
  x_dq : Inport
  Demux : Demux  Outputs=2
  Real-Imag to Complex : RealImagToComplex
  x_d+ix_q : Outport
  wires:
  Demux/1 -> Real-Imag to Complex/1
  Demux/2 -> Real-Imag to Complex/2
  x_dq/1 -> Demux/1
  Real-Imag to Complex/1 -> x_d+ix_q/1

== system WF_offshore/WT_MF14/Control System/Current controller/Subsystem1/Subsystem6 ==
  x_d+ix_q : Inport
  Complex to Real-Imag2 : ComplexToRealImag
  Mux : Mux  Inputs=2
  x_dq : Outport
  wires:
  Complex to Real-Imag2/1 -> Mux/1
  Complex to Real-Imag2/2 -> Mux/2
  Mux/1 -> x_dq/1
  x_d+ix_q/1 -> Complex to Real-Imag2/1

== system WF_offshore/WT_MF2/Control System/Current controller/Subsystem1/Subsystem3 ==
  x_dq : Inport
  Demux : Demux  Outputs=2
  Real-Imag to Complex : RealImagToComplex
  x_d+ix_q : Outport
  wires:
  Real-Imag to Complex/1 -> x_d+ix_q/1
  x_dq/1 -> Demux/1
  Demux/2 -> Real-Imag to Complex/2
  Demux/1 -> Real-Imag to Complex/1

== system WF_offshore/WT_MF2/Control System/Current controller/Subsystem1/Subsystem6 ==
  x_d+ix_q : Inport
  Complex to Real-Imag2 : ComplexToRealImag
  Mux : Mux  Inputs=2
  x_dq : Outport
  wires:
  x_d+ix_q/1 -> Complex to Real-Imag2/1
  Mux/1 -> x_dq/1
  Complex to Real-Imag2/2 -> Mux/2
  Complex to Real-Imag2/1 -> Mux/1

== system WF_offshore/WT_MF3/Control System/Current controller/Subsystem1/Subsystem3 ==
  x_dq : Inport
  Demux : Demux  Outputs=2
  Real-Imag to Complex : RealImagToComplex
  x_d+ix_q : Outport
  wires:
  Demux/1 -> Real-Imag to Complex/1
  Demux/2 -> Real-Imag to Complex/2
  x_dq/1 -> Demux/1
  Real-Imag to Complex/1 -> x_d+ix_q/1

== system WF_offshore/WT_MF3/Control System/Current controller/Subsystem1/Subsystem6 ==
  x_d+ix_q : Inport
  Complex to Real-Imag2 : ComplexToRealImag
  Mux : Mux  Inputs=2
  x_dq : Outport
  wires:
  Complex to Real-Imag2/1 -> Mux/1
  Complex to Real-Imag2/2 -> Mux/2
  Mux/1 -> x_dq/1
  x_d+ix_q/1 -> Complex to Real-Imag2/1

== system WF_offshore/WT_MF4/Control System/Current controller/Subsystem1/Subsystem3 ==
  x_dq : Inport
  Demux : Demux  Outputs=2
  Real-Imag to Complex : RealImagToComplex
  x_d+ix_q : Outport
  wires:
  Real-Imag to Complex/1 -> x_d+ix_q/1
  x_dq/1 -> Demux/1
  Demux/2 -> Real-Imag to Complex/2
  Demux/1 -> Real-Imag to Complex/1

== system WF_offshore/WT_MF4/Control System/Current controller/Subsystem1/Subsystem6 ==
  x_d+ix_q : Inport
  Complex to Real-Imag2 : ComplexToRealImag
  Mux : Mux  Inputs=2
  x_dq : Outport
  wires:
  x_d+ix_q/1 -> Complex to Real-Imag2/1
  Mux/1 -> x_dq/1
  Complex to Real-Imag2/2 -> Mux/2
  Complex to Real-Imag2/1 -> Mux/1

== system WF_offshore/WT_MF5/Control System/Current controller/Subsystem1/Subsystem3 ==
  x_dq : Inport
  Demux : Demux  Outputs=2
  Real-Imag to Complex : RealImagToComplex
  x_d+ix_q : Outport
  wires:
  Demux/1 -> Real-Imag to Complex/1
  Demux/2 -> Real-Imag to Complex/2
  x_dq/1 -> Demux/1
  Real-Imag to Complex/1 -> x_d+ix_q/1

== system WF_offshore/WT_MF5/Control System/Current controller/Subsystem1/Subsystem6 ==
  x_d+ix_q : Inport
  Complex to Real-Imag2 : ComplexToRealImag
  Mux : Mux  Inputs=2
  x_dq : Outport
  wires:
  Complex to Real-Imag2/1 -> Mux/1
  Complex to Real-Imag2/2 -> Mux/2
  Mux/1 -> x_dq/1
  x_d+ix_q/1 -> Complex to Real-Imag2/1

== system WF_offshore/WT_MF6/Control System/Current controller/Subsystem1/Subsystem3 ==
  x_dq : Inport
  Demux : Demux  Outputs=2
  Real-Imag to Complex : RealImagToComplex
  x_d+ix_q : Outport
  wires:
  Real-Imag to Complex/1 -> x_d+ix_q/1
  x_dq/1 -> Demux/1
  Demux/2 -> Real-Imag to Complex/2
  Demux/1 -> Real-Imag to Complex/1

== system WF_offshore/WT_MF6/Control System/Current controller/Subsystem1/Subsystem6 ==
  x_d+ix_q : Inport
  Complex to Real-Imag2 : ComplexToRealImag
  Mux : Mux  Inputs=2
  x_dq : Outport
  wires:
  x_d+ix_q/1 -> Complex to Real-Imag2/1
  Mux/1 -> x_dq/1
  Complex to Real-Imag2/2 -> Mux/2
  Complex to Real-Imag2/1 -> Mux/1

== system WF_offshore/WT_MF7/Control System/Current controller/Subsystem1/Subsystem3 ==
  x_dq : Inport
  Demux : Demux  Outputs=2
  Real-Imag to Complex : RealImagToComplex
  x_d+ix_q : Outport
  wires:
  Demux/1 -> Real-Imag to Complex/1
  Demux/2 -> Real-Imag to Complex/2
  x_dq/1 -> Demux/1
  Real-Imag to Complex/1 -> x_d+ix_q/1

== system WF_offshore/WT_MF7/Control System/Current controller/Subsystem1/Subsystem6 ==
  x_d+ix_q : Inport
  Complex to Real-Imag2 : ComplexToRealImag
  Mux : Mux  Inputs=2
  x_dq : Outport
  wires:
  Complex to Real-Imag2/1 -> Mux/1
  Complex to Real-Imag2/2 -> Mux/2
  Mux/1 -> x_dq/1
  x_d+ix_q/1 -> Complex to Real-Imag2/1

== system WF_offshore/WT_MF8/Control System/Current controller/Subsystem1/Subsystem3 ==
  x_dq : Inport
  Demux : Demux  Outputs=2
  Real-Imag to Complex : RealImagToComplex
  x_d+ix_q : Outport
  wires:
  Real-Imag to Complex/1 -> x_d+ix_q/1
  x_dq/1 -> Demux/1
  Demux/2 -> Real-Imag to Complex/2
  Demux/1 -> Real-Imag to Complex/1

== system WF_offshore/WT_MF8/Control System/Current controller/Subsystem1/Subsystem6 ==
  x_d+ix_q : Inport
  Complex to Real-Imag2 : ComplexToRealImag
  Mux : Mux  Inputs=2
  x_dq : Outport
  wires:
  x_d+ix_q/1 -> Complex to Real-Imag2/1
  Mux/1 -> x_dq/1
  Complex to Real-Imag2/2 -> Mux/2
  Complex to Real-Imag2/1 -> Mux/1

== system WF_offshore/WT_MF9/Control System/Current controller/Subsystem1/Subsystem3 ==
  x_dq : Inport
  Demux : Demux  Outputs=2
  Real-Imag to Complex : RealImagToComplex
  x_d+ix_q : Outport
  wires:
  Demux/1 -> Real-Imag to Complex/1
  Demux/2 -> Real-Imag to Complex/2
  x_dq/1 -> Demux/1
  Real-Imag to Complex/1 -> x_d+ix_q/1

== system WF_offshore/WT_MF9/Control System/Current controller/Subsystem1/Subsystem6 ==
  x_d+ix_q : Inport
  Complex to Real-Imag2 : ComplexToRealImag
  Mux : Mux  Inputs=2
  x_dq : Outport
  wires:
  Complex to Real-Imag2/1 -> Mux/1
  Complex to Real-Imag2/2 -> Mux/2
  Mux/1 -> x_dq/1
  x_d+ix_q/1 -> Complex to Real-Imag2/1
